simulink model "MdBsyClear6s7s"  (R2024b)
settings: Solver=FixedStepDiscrete  StartTime=0.0  StopTime=10.0  FixedStep=0.01  RelTol=1e-3
undefined symbols (not defined in the file or in its folder): ClearBit, IsStBsy32_Clear
settings Model: Creator=sn2xws  LastModifiedBy=sn55gm
settings Model: ModifiedHistory=|
  | 2024.7.11 V3.0.0 557模式流程V1.9
  | 2024.9.2 V3.0.1 最新共存需求V3.0.1
  | 2024.9/26 V3.0.2 计算优先级有问题，增加括号
  | 2024.9.30 V3.0.3 Md30 Md31 清bsy逻辑变更
  | 2024.12.18 V3.0.4 增加Md57 Md58清bsy逻辑
  | 2024.12.25 V3.0.5 Md57 Md58连线未连上问题,增加Md56大四座清bsy逻辑
settings SolverCC: AlgebraicLoopSolver=TrustRegion
settings DataIOCC: SaveFormat=StructureWithTime  ReturnWorkspaceOutputs=off
settings OptimizationCC: DefaultParameterBehavior=Inlined  EnhancedBackFolding=on  PassReuseOutputArgsAs=Individual arguments  ZeroExternalMemoryAtStartup=off  ZeroInternalMemoryAtStartup=off  OptimizeBlockOrder=speed  DifferentSizesBufferReuse=on  OptimizationCustomize=off  EfficientTunableParamExpr=on
settings DebuggingCC: ParameterTunabilityLossMsg=error  UnconnectedInputMsg=warning  UnconnectedOutputMsg=warning  UnconnectedLineMsg=warning  ArithmeticOperatorsInVariantConditions=warning
settings ModelReferenceCC: EnableRefExpFcnMdlSchedulingChecks=on  ModelReferenceNumInstancesAllowed=Single
settings SFSimCC: MATLABDynamicMemAlloc=off  CustomCodeUndefinedFunction=UseInterfaceOnly
settings RTWCC: Description=AUTOSAR  SystemTargetFile=autosar.tlc  GenCodeOnly=on  TemplateMakefile=ert_default_tmf  GenerateReport=on  IncludeHyperlinkInReport=on  LaunchReport=on  DataTypeReplacement=CDataTypesFixedWidth  GenerateTraceInfo=on  GenerateTraceReport=on  GenerateTraceReportSl=on  GenerateTraceReportSf=on  GenerateTraceReportEml=on  GenerateCodeMetricsReport=on  GPUComputeCapability=3.5
settings CodeAppCC: ForceParamTrailComments=on  IgnoreCustomStorageClasses=off  OperatorAnnotations=on  SimulinkDataObjDesc=on  SFDataObjDesc=on  InsertBlockDesc=on
settings STFCustomTargetCC: TargetLangStandard=C99 (ISO)  MultiwordLength=256  ParMdlRefBuildCompliant=on  CompOptLevelCompliant=on  IncludeMdlTerminateFcn=off  CombineOutputUpdateFcns=on  SuppressErrorStatus=on  ERTCustomFileBanners=on  SupportNonFinite=off  SupportComplex=off  SupportContinuousTime=off  SupportNonInlinedSFcns=off  RemoveResetFunc=on  MATLABClassNameForMDSCustomization=Simulink.SoftwareTarget.ERTCustomization  AutosarCompliant=on  UseToolchainInfoCompliant=on  LookupTableObjectStructAxisOrder=2,1,3,4,...  LUTObjectStructOrderEvenSpacing=Size,Table,Breakpoints  SystemTargetFile=autosar.tlc
settings ERTTargetCC: TargetLangStandard=C99 (ISO)  ConcurrentExecutionCompliant=off  IncludeMdlTerminateFcn=off  SuppressErrorStatus=on  SupportNonFinite=off  SupportComplex=off  ModelStepFunctionPrototypeControlCompliant=off  CPPClassGenCompliant=off  AutosarCompliant=on  LookupTableObjectStructAxisOrder=2,1,3,4,...  LUTObjectStructOrderEvenSpacing=Size,Table,Breakpoints  ERTCustomFileTemplate=example_file_process.tlc  ERTFilePackagingFormat=Compact  BooleanTrueId=TRUE  BooleanFalseId=FALSE  DynamicArrayContainerType=coder::array

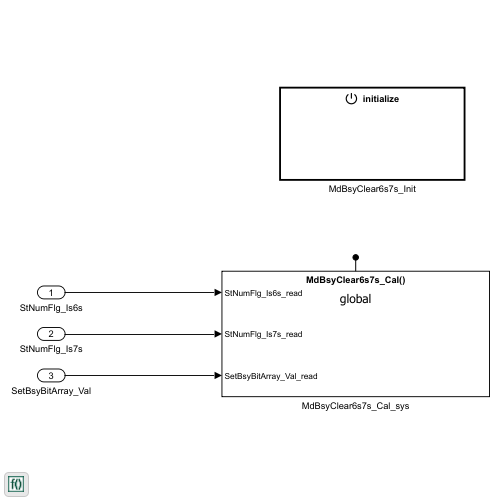
[thumbnail: Simulink's stored preview of the top-level diagram]
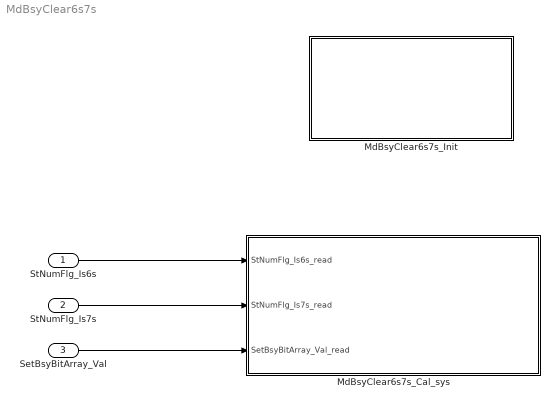
== system MdBsyClear6s7s ==
  StNumFlg_Is6s : Inport  OutDataTypeStr=boolean  PortDimensions=1
  StNumFlg_Is7s : Inport  Port=2  OutDataTypeStr=boolean  PortDimensions=1
  SetBsyBitArray_Val : Inport  Port=3  OutDataTypeStr=uint32  PortDimensions=32
  MdBsyClear6s7s_Cal_sys : Subsystem
  MdBsyClear6s7s_Init : Subsystem
  wires:
  StNumFlg_Is6s/1 -> MdBsyClear6s7s_Cal_sys/1(StNumFlg_Is6s_read)
  StNumFlg_Is7s/1 -> MdBsyClear6s7s_Cal_sys/2(StNumFlg_Is7s_read)
  SetBsyBitArray_Val/1 -> MdBsyClear6s7s_Cal_sys/3(SetBsyBitArray_Val_read)

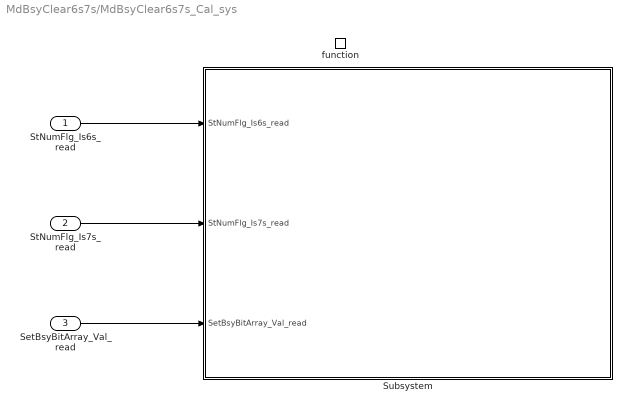
== system MdBsyClear6s7s/MdBsyClear6s7s_Cal_sys ==
  StNumFlg_Is6s_read : Inport
  StNumFlg_Is7s_read : Inport  Port=2
  SetBsyBitArray_Val_read : Inport  Port=3
  function : TriggerPort  TriggerType=function-call  IsSimulinkFunction=on  FunctionName=MdBsyClear6s7s_Cal  VariantControl=(inherit)
  Subsystem : Subsystem
  wires:
  StNumFlg_Is6s_read/1 -> Subsystem/1(StNumFlg_Is6s_read)
  StNumFlg_Is7s_read/1 -> Subsystem/2(StNumFlg_Is7s_read)
  SetBsyBitArray_Val_read/1 -> Subsystem/3(SetBsyBitArray_Val_read)

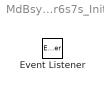
== system MdBsyClear6s7s/MdBsyClear6s7s_Init ==
  Event Listener : EventListener  EventName=reset

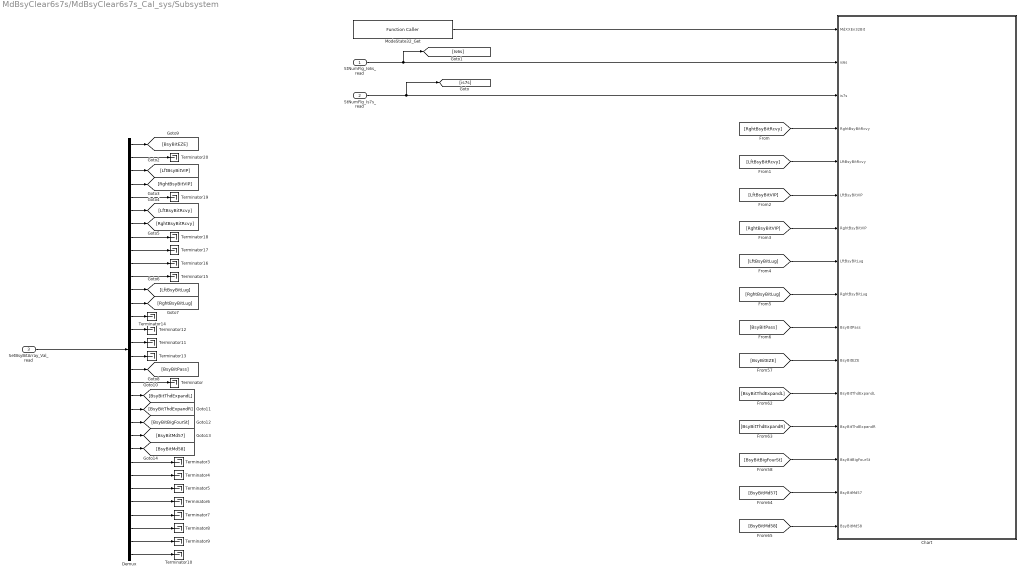
== system MdBsyClear6s7s/MdBsyClear6s7s_Cal_sys/Subsystem ==
  StNumFlg_Is6s_read : Inport
  StNumFlg_Is7s_read : Inport  Port=2
  SetBsyBitArray_Val_read : Inport  Port=3
  Chart : Stateflow chart  TreatAsAtomicUnit=on
  Demux : Demux  Outputs=32
  ModeState32_Get : FunctionCaller  FunctionPrototype=MdEn32 = ModeState32_Get()  InputArgumentSpecifications=<Enter example>  OutputArgumentSpecifications=uint32(1)
  Terminator{,3..20} (19 alike) : Terminator
  wires:
  StNumFlg_Is6s_read/1 -> [Is6s], Chart/2(is6s)
  StNumFlg_Is7s_read/1 -> [is7s], Chart/3(is7s)
  ModeState32_Get/1 -> Chart/1(MdXXEn32Bit)
  [RghtBsyBitRcvy] -> Chart/4(RghtBsyBitRcvy)
  [LftBsyBitRcvy] -> Chart/5(LftBsyBitRcvy)
  [LftBsyBitVIP] -> Chart/6(LftBsyBitVIP)
  [RghtBsyBitVIP] -> Chart/7(RghtBsyBitVIP)
  [LftBsyBitLug] -> Chart/8(LftBsyBitLug)
  [RghtBsyBitLug] -> Chart/9(RghtBsyBitLug)
  [BsyBitPass] -> Chart/10(BsyBitPass)
  SetBsyBitArray_Val_read/1 -> Demux/1
  Demux/3 -> [LftBsyBitVIP]
  Demux/4 -> [RghtBsyBitVIP]
  Demux/6 -> [LftBsyBitRcvy]
  Demux/7 -> [RghtBsyBitRcvy]
  Demux/12 -> [LftBsyBitLug]
  Demux/13 -> [RghtBsyBitLug]
  Demux/18 -> [BsyBitPass]
  Demux/19 -> Terminator/1
  Demux/23 -> [BsyBitMd57]
  Demux/24 -> [BsyBitMd58]
  Demux/25 -> Terminator3/1
  Demux/26 -> Terminator4/1
  Demux/27 -> Terminator5/1
  Demux/28 -> Terminator6/1
  Demux/29 -> Terminator7/1
  Demux/30 -> Terminator8/1
  Demux/31 -> Terminator9/1
  Demux/32 -> Terminator10/1
  Demux/16 -> Terminator11/1
  Demux/15 -> Terminator12/1
  Demux/17 -> Terminator13/1
  Demux/14 -> Terminator14/1
  Demux/1 -> [BsyBitEZE]
  Demux/20 -> [BsyBitThdExpandL]
  Demux/21 -> [BsyBitThdExpandR]
  Demux/22 -> [BsyBitBigFourSt]
  [BsyBitBigFourSt] -> Chart/14(BsyBitBigFourSt)
  [BsyBitThdExpandR] -> Chart/13(BsyBitThdExpandR)
  [BsyBitThdExpandL] -> Chart/12(BsyBitThdExpandL)
  [BsyBitEZE] -> Chart/11(BsyBitEZE)
  Demux/11 -> Terminator15/1
  Demux/10 -> Terminator16/1
  Demux/9 -> Terminator17/1
  Demux/8 -> Terminator18/1
  Demux/5 -> Terminator19/1
  Demux/2 -> Terminator20/1
  [BsyBitMd58] -> Chart/16(BsyBitMd58)
  [BsyBitMd57] -> Chart/15(BsyBitMd57)

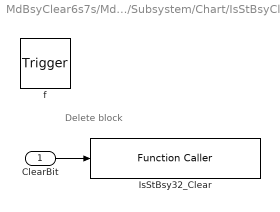
== system MdBsyClear6s7s/MdBsyClear6s7s_Cal_sys/Subsystem/Chart/IsStBsyClear ==
  note: Delete block
  ClearBit : Inport
  f : TriggerPort  TriggerType=function-call  VariantControl=(inherit)
      settings: CopyFcn=Stateflow.SLINSF.SimulinkMan.removeBlockPreDeleteFcn  PreDeleteFcn=Stateflow.SLINSF.SimulinkMan.unsafePredeleteFcn
  IsStBsy32_Clear : FunctionCaller  FunctionPrototype=IsStBsy32_Clear(ClearBit)  InputArgumentSpecifications=uint32(1)  OutputArgumentSpecifications=<Enter example>
  wires:
  ClearBit/1 -> IsStBsy32_Clear/1

== stateflow chart MdBsyClear6s7s/MdBsyClear6s7s_Cal_sys/Subsystem/Chart ==
  state IsStBsyClear(ClearBit) [function]
  (default) -> (junction 13) : {
      | //AllMdBit = EZEBit+VIPAllBit+LugAllBit+VIPExitAllBit+Md56Bit;
      | //LftMdBit6s7s = VIPLBit+RcvyLBit + LugLBit;
      | //RghtMdBit6s7s =  VIPRBit+RcvyRBit + LugRBit;
      | ClearBit = 0;
      | }
  (junction 13) -> (junction 2)
  (junction 2) -> (junction 27) [order 1] : [MdXXEn32Bit ==0]
  (junction 2) -> (junction 1) [order 2]
  (junction 27) -> (junction 40) : {ClearBit = 4294967295;}
  (junction 1) -> (junction 110) [order 1] : [(MdXXEn32Bit &RghtBsyBitRcvy) == 0]
  (junction 1) -> (junction 114) [order 2]
  (junction 110) -> (junction 112) : {ClearBit =RcvyRBit; }
  (junction 112) -> (junction 114)
  (junction 114) -> (junction 19)
  (junction 19) -> (junction 17) [order 1] : [(MdXXEn32Bit &LftBsyBitRcvy)==0]
  (junction 19) -> (junction 3) [order 2]
  (junction 17) -> (junction 18) : {ClearBit =  ((ClearBit+RcvyLBit));}
  (junction 18) -> (junction 3)
  (junction 3) -> (junction 4)
  (junction 4) -> (junction 5) [order 1] : [(MdXXEn32Bit &LftBsyBitVIP)==0]
  (junction 4) -> (junction 6) [order 2]
  (junction 5) -> (junction 15) : {ClearBit = ClearBit +VIPLBit+VIPLExitBit+0x2000;}
  (junction 15) -> (junction 6)
  (junction 6) -> (junction 118)
  (junction 118) -> (junction 120) [order 1] : [(MdXXEn32Bit &RghtBsyBitVIP)==0]
  (junction 118) -> (junction 20) [order 2]
  (junction 120) -> (junction 122) : {ClearBit = ClearBit +VIPRBit+VIPRExitBit+0x4000;}
  (junction 122) -> (junction 20)
  (junction 20) -> (junction 125)
  (junction 125) -> (junction 127) [order 1] : [(MdXXEn32Bit &LftBsyBitLug)==0]
  (junction 125) -> (junction 131) [order 2]
  (junction 127) -> (junction 129) : {ClearBit = ClearBit +LugLBit;}
  (junction 129) -> (junction 131)
  (junction 131) -> (junction 9)
  (junction 9) -> (junction 10) [order 1] : [(MdXXEn32Bit &RghtBsyBitLug)==0]
  (junction 9) -> (junction 11) [order 2]
  (junction 10) -> (junction 16) : {ClearBit = ClearBit +LugRBit;}
  (junction 16) -> (junction 11)
  (junction 11) -> (junction 143)
  (junction 143) -> (junction 152) [order 1] : [(MdXXEn32Bit &BsyBitThdExpandL)==0]
  (junction 143) -> (junction 149) [order 2]
  (junction 152) -> (junction 154) : {ClearBit = ClearBit +Md32Bit;}
  (junction 154) -> (junction 149)
  (junction 149) -> (junction 161)
  (junction 161) -> (junction 163) [order 1] : [(MdXXEn32Bit &BsyBitThdExpandR)==0]
  (junction 161) -> (junction 167) [order 2]
  (junction 163) -> (junction 165) : {ClearBit = ClearBit +Md53Bit;}
  (junction 165) -> (junction 167)
  (junction 167) -> (junction 138)
  (junction 138) -> (junction 22) [order 1] : [(MdXXEn32Bit &BsyBitPass)==0]
  (junction 138) -> (junction 24) [order 2]
  (junction 22) -> (junction 59) : {ClearBit = ClearBit +Md30Bit+Md31Bit;}
  (junction 59) -> (junction 24)
  (junction 24) -> (junction 183)
  (junction 183) -> (junction 185) [order 1] : [(MdXXEn32Bit &BsyBitMd57)==0]
  (junction 183) -> (junction 190) [order 2]
  (junction 185) -> (junction 188) : {ClearBit = ClearBit +Md57Bit+Md58Bit;}
  (junction 188) -> (junction 190)
  (junction 190) -> (junction 197)
  (junction 197) -> (junction 199) [order 1] : [(MdXXEn32Bit &BsyBitBigFourSt)==0]
  (junction 197) -> (junction 203) [order 2]
  (junction 199) -> (junction 201) : {ClearBit = ClearBit + Md56Bit;}
  (junction 201) -> (junction 203)
  (junction 203) -> (junction 206)
  (junction 206) -> (junction 208) [order 1] : [(MdXXEn32Bit &BsyBitEZE)==0]
  (junction 206) -> (junction 212) [order 2]
  (junction 208) -> (junction 210) : {ClearBit = ClearBit +EZEBit;}
  (junction 210) -> (junction 212)
  (junction 212) -> (junction 194)
  (junction 40) -> (junction 194)
  (junction 194) -> (junction 94) : {
      | IsStBsyClear(ClearBit);
      | }
  data: ClearBit function_input; MdXXEn32Bit input uint32; is6s input boolean; is7s input boolean; EZEBit constant uint32 =1; EZQBit constant uint32 =8; VIPAllBit constant uint32 =2; LugAllBit constant uint32 =4; VIPLBit constant uint32 =512; VIPRBit constant uint32 =2048; RcvyLBit constant uint32 =1024; RcvyRBit constant uint32 =4096; INTMLBit constant uint32 =16; INTMRBit constant uint32 =524288; FamlyLBit constant uint32 =64; FamlyRBit constant uint32 =32; LugLBit constant uint32 =128; LugRBit constant uint32 =256; LftMdBit6s7s local uint32; AllMdBit local uint32; RghtMdBit6s7s local uint32; ClearBit local uint32; VIPLExitBit constant uint32 =67108864; VIPRExitBit constant uint32 =134217728; VIPExitAllBit constant uint32 =268435456; Md32Bit constant uint32 =2147483648; Md53Bit constant uint32 =131072; RghtBsyBitRcvy input uint32; LftBsyBitRcvy input uint32; LftBsyBitVIP input uint32; RghtBsyBitVIP input uint32; LftBsyBitLug input uint32; RghtBsyBitLug input uint32; BsyBitPass input uint32; Md30Bit constant uint32 =536870912; Md31Bit constant uint32 =1073741824; Md56Bit constant uint32 =16777216; BsyBitEZE input uint32; BsyBitThdExpandL input uint32; BsyBitThdExpandR input uint32; BsyBitBigFourSt input uint32; BsyBitMd57 input uint32; BsyBitMd58 input uint32; Md57Bit constant uint32 =1048576; Md58Bit constant uint32 =2097152; BedLBit constant uint32 =8192; BedRBit constant uint32 =16384
